simulink model "BevraniAGC2"  (Simulink 7.9)
settings: Solver=ode45  StartTime=0.0  StopTime=600  RelTol=1e-3
InitFcn:
  | BevraniAGC3_init
values from neighbouring files (symbols this model uses):
  B1 = 0.3483    [BevraniAGC3_init.m]
  B2 = 0.3827    [BevraniAGC3_init.m]
  D1 = 0.015    [BevraniAGC3_init.m]
  D2 = 0.016    [BevraniAGC3_init.m]
  H1 = 0.1667/2    (= 0.08335)    [BevraniAGC3_init.m]
  H2 = 0.2017/2    (= 0.10085)    [BevraniAGC3_init.m]
  R1 = 3.00    (= 3)    [BevraniAGC3_init.m]
  R2 = 2.73    [BevraniAGC3_init.m]
  T12 = 0.20    (= 0.2)    [BevraniAGC3_init.m]
  Tg1 = 0.08    [BevraniAGC3_init.m]
  Tg2 = 0.06    [BevraniAGC3_init.m]
  Tt1 = 0.40    (= 0.4)    [BevraniAGC3_init.m]
  Tt2 = 0.44    [BevraniAGC3_init.m]
undefined symbols (not defined in the file or in its folder): K1, K2, UFLS
libraries: powerlib x1
settings Model: Creator=ywlaw  LastModifiedBy=ywlaw
settings DebuggingCC: SolverPrmCheckMsg=none
settings GRTTargetCC: CombineOutputUpdateFcns=off  GRTInterface=on

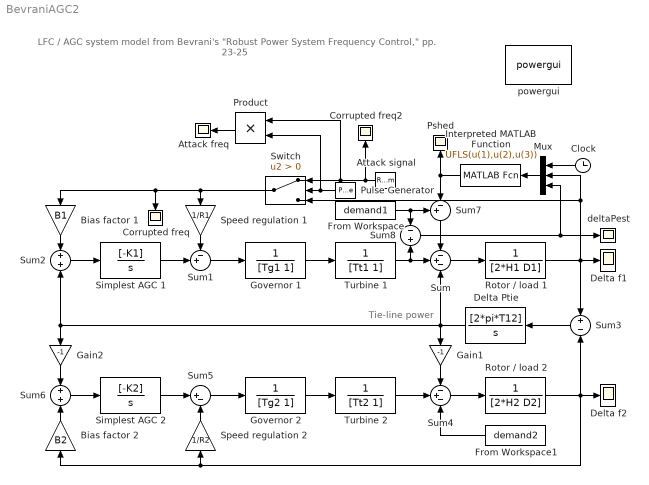
== system BevraniAGC2 ==
  note: LFC / AGC system model from Bevrani's "Robust Power System Frequency Control," pp. 23-25
  note: Tie-line power
  Attack freq : Scope
      settings: TimeRange=20  YMin=-4  YMax=1  SaveName=attackFreq
  Attack signal : UniformRandomNumber  Minimum=-3  Maximum=-0.5  Seed=1234  SampleTime=60
  Bias factor 1 : Gain  Gain=B1
  Bias factor 2 : Gain  Gain=B2
  Clock : Clock
  Corrupted freq : Scope
      settings: TimeRange=20  YMin=-4  YMax=1  SaveName=corruptedFreq
  Corrupted freq2 : Scope
      settings: TimeRange=20  YMin=-4  YMax=1  SaveName=attackfreq1
  Delta Ptie : TransferFcn  Numerator=[2*pi*T12]  Denominator=[1 0]
  Delta f1 : Scope
      settings: TimeRange=30  YMin=-0.002  YMax=0.014  SaveName=deltaf1
  Delta f2 : Scope
      settings: TimeRange=20
  From Workspace : FromWorkspace  VariableName=demand1  SampleTime=5
  From Workspace1 : FromWorkspace  VariableName=demand2  SampleTime=5
  Gain1 : Gain  Gain=-1
  Gain2 : Gain  Gain=-1
  Governor 1 : TransferFcn  Denominator=[Tg1 1]
  Governor 2 : TransferFcn  Denominator=[Tg2 1]
  Interpreted MATLAB Function : MATLABFcn  MATLABFcn=UFLS(u(1),u(2),u(3))  SampleTime=0.05
  Mux : Mux  Inputs=3
  Product : Product  RndMeth=Zero
  Pshed : Scope
      settings: TimeRange=20  YMin=-4  YMax=1  SaveName=Pshed
  Pulse Generator : DiscretePulseGenerator  PulseType=Time based  Period=60  PulseWidth=10  PhaseDelay=100
  Rotor / load 1 : TransferFcn  Denominator=[2*H1 D1]
  Rotor / load 2 : TransferFcn  Denominator=[2*H2 D2]
  Simplest AGC 1 : TransferFcn  Numerator=[-K1]  Denominator=[1 0]
  Simplest AGC 2 : TransferFcn  Numerator=[-K2]  Denominator=[1 0]
  Speed regulation 1 : Gain  Gain=1/R1
  Speed regulation 2 : Gain  Gain=1/R2
  Sum : Sum  Inputs=-+-
  Sum1 : Sum  Inputs=-+|
  Sum2 : Sum  Inputs=+|+
  Sum3 : Sum  Inputs=+|-
  Sum4 : Sum  Inputs=-+-
  Sum5 : Sum  Inputs=|+-
  Sum6 : Sum  Inputs=+|+
  Sum7 : Sum  Inputs=+-|
  Sum8 : Sum  Inputs=-|+
  Switch : Switch  Criteria=u2 > Threshold  SampleTime=0.1
  Turbine 1 : TransferFcn  Denominator=[Tt1 1]
  Turbine 2 : TransferFcn  Denominator=[Tt2 1]
  deltaPest : Scope
      settings: TimeRange=20  YMin=-4  YMax=1  SaveName=deltaPest
  powergui : powerlib/powergui  Priority=1  SimulationMode=Continuous  SolverType=Tustin  SampleTime=50e-6  frequency=60  SPID=off  DisableSnubberDevices=off  DisableRonSwitches=off  DisableVfSwitches=off  SwTol=0  Interpol=off  DisplayEquations=off  FunctionMessages=off  frequencyindice=60  Pbase=100e6  ErrMax=1e-4  Iterations=50  UnitsV=kV  UnitsW=MW  echomessages=off  HookPort=off  EnableUseOfTLC=off  x0status=blocks  RestoreLinks=warning  ResistiveCurrentMeasurement=off  Ylog=off  Xlog=on  ShowGrid=off  save=off  variable=ZData  ZoomFFT=off  StartTime=0.0  cycles=1  DisplayStyle=1  FreqAxis=off  MaxFrequency=1000  frequencyindicesteady=1  display=off  methode=off
  wires:
  Turbine 1/1 -> Sum/2, Sum8/2
  Governor 1/1 -> Turbine 1/1
  Sum/1 -> Rotor / load 1/1
  Sum1/1 -> Governor 1/1
  Rotor / load 1/1 -> Delta f1/1, Sum3/1, Switch/3, Mux/2
  Speed regulation 1/1 -> Sum1/1
  Simplest AGC 1/1 -> Sum1/2
  Sum3/1 -> Delta Ptie/1
  Bias factor 1/1 -> Sum2/1
  Sum2/1 -> Simplest AGC 1/1
  Turbine 2/1 -> Sum4/2
  Governor 2/1 -> Turbine 2/1
  Sum4/1 -> Rotor / load 2/1
  Sum5/1 -> Governor 2/1
  Rotor / load 2/1 -> Delta f2/1, Sum3/2, Speed regulation 2/1, Bias factor 2/1
  Sum6/1 -> Simplest AGC 2/1
  Simplest AGC 2/1 -> Sum5/1
  Speed regulation 2/1 -> Sum5/2
  Bias factor 2/1 -> Sum6/2
  Gain1/1 -> Sum4/1
  Delta Ptie/1 -> Sum/3, Gain1/1, Sum2/2, Gain2/1
  Gain2/1 -> Sum6/1
  From Workspace1/1 -> Sum4/3
  Pulse Generator/1 -> Switch/2, Product/2
  Switch/1 -> Speed regulation 1/1, Bias factor 1/1, Corrupted freq/1
  Attack signal/1 -> Switch/1, Product/1, Corrupted freq2/1
  Product/1 -> Attack freq/1
  Sum7/1 -> Sum/1
  Mux/1 -> Interpreted MATLAB Function/1
  Clock/1 -> Mux/1
  From Workspace/1 -> Sum7/1, Sum8/1
  Sum8/1 -> Mux/3, deltaPest/1
  Interpreted MATLAB Function/1 -> Sum7/2, Pshed/1
